simulink model "JumpingHalfLekaSpeedgoat30cm"  (R2024a)
settings: Solver=FixedStepAuto  StartTime=0.0  StopTime=inf  RelTol=1e-3
undefined symbols (not defined in the file): HS, IO291
libraries: aru_toolbox x6, speedgoatlib_IO691 x1, speedgoatlib_IO291 x1, simulink x1
settings Model: Creator=Blue Fifth  LastModifiedBy=user
settings SolverCC: ConcurrentTasks=on  PositivePriorityOrder=on  AutoInsertRateTranBlk=on
settings OptimizationCC: BlockReduction=off  OptimizeBlockIOStorage=off
settings DebuggingCC: TasksWithSamePriorityMsg=none
settings HardwareCC: ProdBitPerLong=64  ProdLongLongMode=on  ProdHWDeviceType=Intel->x86-64 (Linux 64)
settings RTWCC: Description=Speedgoat Real-Time Target Machine  SystemTargetFile=speedgoat.tlc  TemplateMakefile=slrealtime_default_tmf  Toolchain=Simulink Real-Time Toolchain  BuildConfiguration=Faster Runs  CodeExecutionProfiling=on  TargetLang=C++  GPUComputeCapability=3.5
settings SimulinkRealTimeTargetCC: InstructionSetFMA=off  LogToMDFFile=off

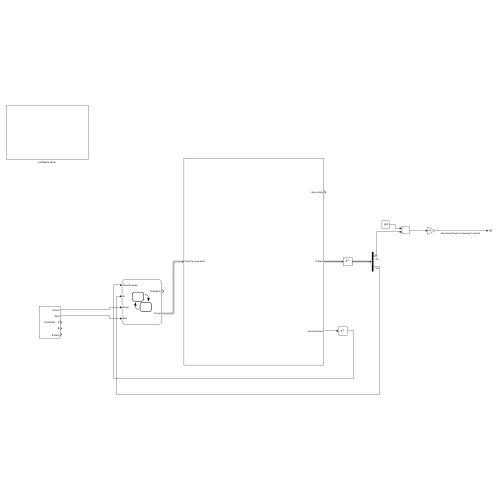
[thumbnail: Simulink's stored preview of the top-level diagram]
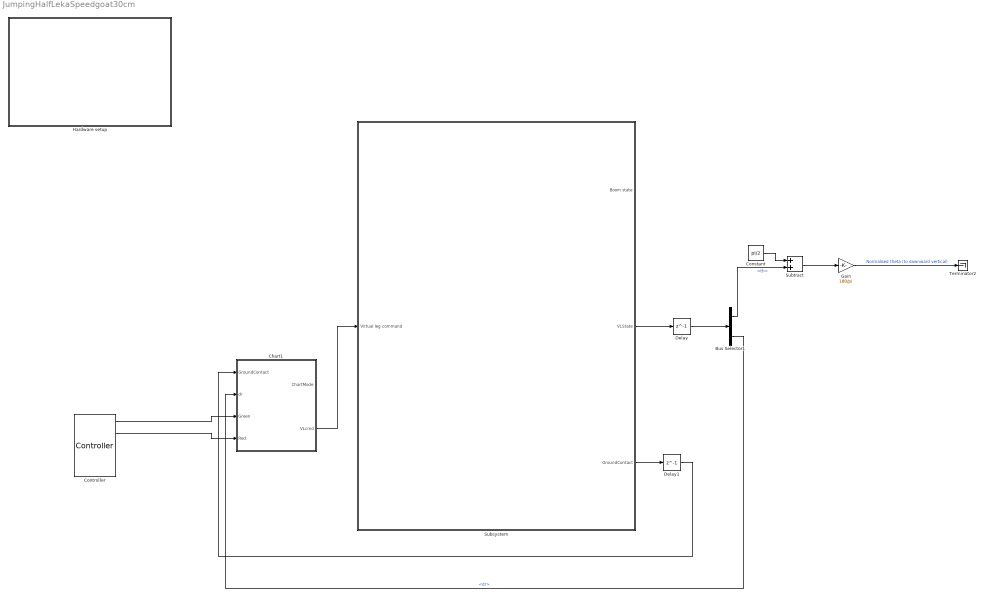
== system JumpingHalfLekaSpeedgoat30cm ==
  Bus Selector1 : BusSelector  OutputSignals=th,dr
  Chart1 : Stateflow chart  TreatAsAtomicUnit=on
  Constant : Constant  Value=pi/2
  Controller : aru_toolbox/Controller
      settings: SourceProductName=ARU Toolbox
  Delay : Delay  DelayLength=1
  Delay1 : Delay  DelayLength=1
  Gain : Gain  Gain=180/pi
  Hardware setup : Subsystem
  Subsystem : Subsystem
  Subtract : Sum
  Terminator2 : Terminator
  wires:
  Controller/1 -> Chart1/3(Green)
  Chart1/2(VLcmd) -> Subsystem/1(Virtual leg command)
  Controller/2 -> Chart1/4(Red)
  Delay1/1 -> Chart1/1(GroundContact)
  Subsystem/2(VLState) -> Delay/1
  Bus Selector1/2 -> Chart1/2(dr)  "<dr>"
  Constant/1 -> Subtract/1
  Subtract/1 -> Gain/1
  Gain/1 -> Terminator2/1  "Normalised theta (to downward vertical)"
  Bus Selector1/1 -> Subtract/2  "<th>"
  Delay/1 -> Bus Selector1/1
  Subsystem/3(GroundContact) -> Delay1/1

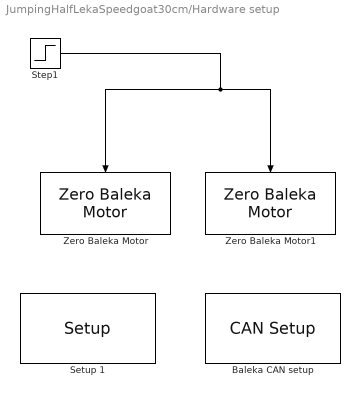
== system JumpingHalfLekaSpeedgoat30cm/Hardware setup ==
  Baleka CAN setup : speedgoatlib_IO691/Legacy/CAN Setup   moduletype=IO691  id=1  pciSlot=-1  chn1=CAN (HS)  chn2=CAN (HS)  chn3=Disabled  chn4=Disabled  initStruct=[]  termStruct=[struct('Channel',1,'Protocol','CAN','BRS',0,'Type','Extended','Identifier',1,'Data',[255, 255, 255, 255, 255, 255, 255, 253],'Pause',0.001), struct('Channel',2,'Protocol','CAN','BRS',0,'Type','Standard','Identifier',2,'Data',[255, 255, 255, 255, 255, 255, 255, 253],'Pause',0.001)]  ArbitrationbdrChn1=1.0 MBaud  ArbitrationManbdrChn1=[2,8,31,8]  FdbdrChn1=1.0 MBaud  FdManbdrChn1=[2,8,31,8]  ArbitrationbdrChn2=1.0 MBaud  ArbitrationManbdrChn2=[2,8,31,8]  FdbdrChn2=1.0 MBaud  FdManbdrChn2=[2,8,31,8]  ArbitrationbdrChn3=1.0 MBaud  ArbitrationManbdrChn3=[2,8,31,8]  FdbdrChn3=5.0 MBaud  FdManbdrChn3=[2,2,5,2]  ArbitrationbdrChn4=1.0 MBaud  ArbitrationManbdrChn4=[2,8,31,8]  FdbdrChn4=5.0 MBaud  FdManbdrChn4=[2,2,5,2]  moduleInitValues=[691 1 -1 -1]
      settings: SourceProductName=IO691
  Setup 1 : speedgoatlib_IO291/Setup   parInternalModuleId=1  parPciSlot=-1  parModuleId=1  parModuleType=IO291-HS  parTtlDoChannels=[]  parTtlDoInitValues=1  parTtlDoReset=1  parTtlDiChannels=[1 2 3 4 5]  parIsolDiChannels=[]  parFetDoChannels=[1 2 3 4 5 6]  parFetDoInitValues=0  parFetDoReset=1
      settings: SourceProductName=IO291
  Step1 : Step  Time=0.3  SampleTime=0
  Zero Baleka Motor : aru_toolbox/Baleka 2.5/Zero Baleka Motor  CAN_ID=1  channel=1
      settings: SourceProductName=ARU Toolbox
  Zero Baleka Motor1 : aru_toolbox/Baleka 2.5/Zero Baleka Motor  CAN_ID=2  channel=1
      settings: SourceProductName=ARU Toolbox
  wires:
  Step1/1 -> Zero Baleka Motor1/Trigger, Zero Baleka Motor/Trigger

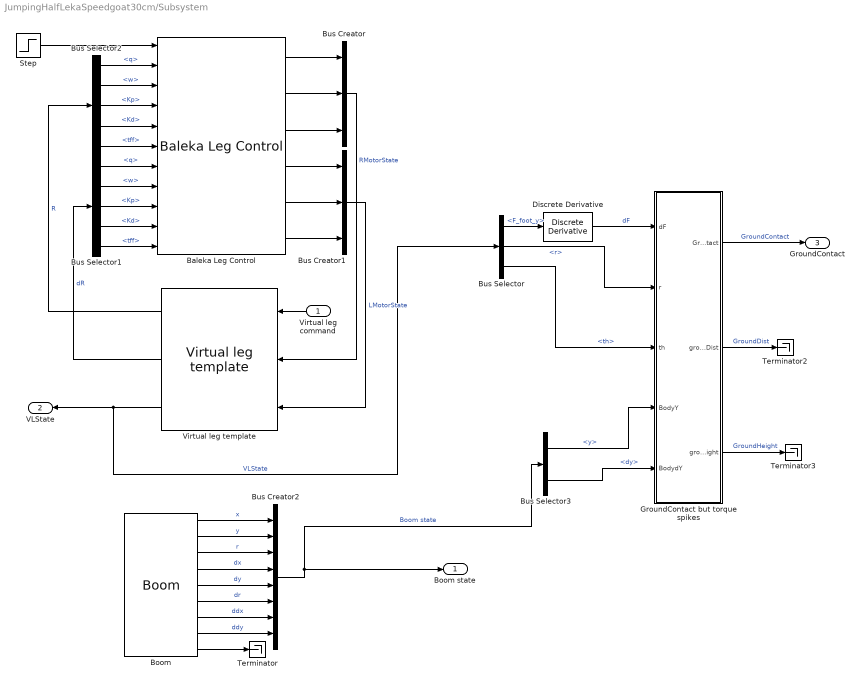
== system JumpingHalfLekaSpeedgoat30cm/Subsystem ==
  Virtual leg command : Inport
  Baleka Leg Control : aru_toolbox/Baleka 2.5/Baleka Leg Control  CAN_ID_L=1  CAN_ID_R=2  channel=1  Comm_freq=1000  enableOffsets=on
      settings: SourceProductName=ARU Toolbox
  Boom : aru_toolbox/Boom  ts=0.001
      settings: SourceProductName=ARU Toolbox
  Bus Creator : BusCreator  Inputs=3  OutDataTypeStr=Bus: MotorState
      settings: InheritFromInputs=off
  Bus Creator1 : BusCreator  Inputs=3  OutDataTypeStr=Bus: MotorState
      settings: InheritFromInputs=off
  Bus Creator2 : BusCreator  Inputs=8  OutDataTypeStr=Bus: BodyState  NonVirtualBus=on
  Bus Selector : BusSelector  OutputSignals=F_foot_y,r,th
  Bus Selector1 : BusSelector  OutputSignals=q,w,Kp,Kd,tff
  Bus Selector2 : BusSelector  OutputSignals=q,w,Kp,Kd,tff
  Bus Selector3 : BusSelector  OutputSignals=y,dy
  Discrete Derivative : simulink/Discrete/Discrete Derivative  gainval=1.0  ICPrevScaledInput=0.0  OutMin=[]  OutMax=[]  OutDataType=fixdt(1, 16)  OutScaling=2^-10  DoSatur=off
  GroundContact but torque spikes : MATLAB Function  TreatAsAtomicUnit=on
  Step : Step  Time=3  SampleTime=0
  Terminator : Terminator
  Terminator2 : Terminator
  Terminator3 : Terminator
  Virtual leg template : aru_toolbox/Baleka 2.5/Virtual leg template  SystemSampleTime=-1  VariantActivationTime=update diagram  AllowFlexibleInterface=on  Latency=0  AutoFrameSizeCalculation=off
      settings: SourceProductName=ARU Toolbox
  Boom state : Outport
  VLState : Outport  Port=2
  GroundContact : Outport  Port=3
  wires:
  Virtual leg template/1 -> Bus Selector2/1  "R"
  Boom/7 -> Bus Creator2/7  "ddx"
  Step/1 -> Baleka Leg Control/1
  Boom/4 -> Bus Creator2/4  "dx"
  Boom/1 -> Bus Creator2/1  "x"
  Boom/2 -> Bus Creator2/2  "y"
  Baleka Leg Control/5 -> Bus Creator1/2
  Bus Selector2/4 -> Baleka Leg Control/5  "<Kd>"
  Baleka Leg Control/3 -> Bus Creator/3
  Boom/6 -> Bus Creator2/6  "dr"
  Baleka Leg Control/2 -> Bus Creator/2
  Baleka Leg Control/6 -> Bus Creator1/3
  Baleka Leg Control/4 -> Bus Creator1/1
  Boom/5 -> Bus Creator2/5  "dy"
  Boom/8 -> Bus Creator2/8  "ddy"
  Bus Selector2/2 -> Baleka Leg Control/3  "<w>"
  Boom/9 -> Terminator/1
  Bus Selector1/1 -> Baleka Leg Control/7  "<q>"
  Bus Selector1/3 -> Baleka Leg Control/9  "<Kp>"
  Bus Creator1/1 -> Virtual leg template/3  "LMotorState"
  Bus Selector1/2 -> Baleka Leg Control/8  "<w>"
  Bus Creator/1 -> Virtual leg template/2  "RMotorState"
  Baleka Leg Control/1 -> Bus Creator/1
  Bus Selector2/1 -> Baleka Leg Control/2  "<q>"
  Virtual leg command/1 -> Virtual leg template/1
  Bus Selector2/3 -> Baleka Leg Control/4  "<Kp>"
  Bus Selector1/4 -> Baleka Leg Control/10  "<Kd>"
  Bus Selector2/5 -> Baleka Leg Control/6  "<tff>"
  Bus Selector1/5 -> Baleka Leg Control/11  "<tff>"
  Boom/3 -> Bus Creator2/3  "r"
  Bus Creator2/1 -> Bus Selector3/1, Boom state/1  "Boom state"
  Virtual leg template/2 -> Bus Selector1/1  "dR"
  Virtual leg template/3 -> Bus Selector/1, VLState/1  "VLState"
  Bus Selector/3 -> GroundContact but torque spikes/3(th)  "<th>"
  Bus Selector3/1 -> GroundContact but torque spikes/4(BodyY)  "<y>"
  Bus Selector3/2 -> GroundContact but torque spikes/5(BodydY)  "<dy>"
  Bus Selector/2 -> GroundContact but torque spikes/2(r)  "<r>"
  Discrete Derivative/1 -> GroundContact but torque spikes/1(dF)  "dF"
  Bus Selector/1 -> Discrete Derivative/1  "<F_foot_y>"
  GroundContact but torque spikes/1(GroundContact) -> GroundContact/1  "GroundContact"
  GroundContact but torque spikes/3(groundHeight) -> Terminator3/1  "GroundHeight"
  GroundContact but torque spikes/2(groundDist) -> Terminator2/1  "GroundDist"

== stateflow chart JumpingHalfLekaSpeedgoat30cm/Chart1 ==
  state Stop
    % Static values
    VLcmd.Tff = 0;
    VLcmd.dth_des =0;
    VLcmd.th_des = -pi/2;
    VLcmd.KPth = 250;
    VLcmd.KDth = 10;
    VLcmd.r_des = 0.45;
    VLcmd.dr_des =0;
    VLcmd.KPr = 1500;
    VLcmd.KDr =50;
    VLcmd.Fff =0;
  state StandUp
    % Static values
    VLcmd.Tff = 0;
    VLcmd.dth_des =0;
    VLcmd.th_des = -pi/2;
    VLcmd.KPth = 50;
    VLcmd.KDth = 5;
    % Gentle stand-up
    VLcmd.r_des = 0.40;
    VLcmd.dr_des =0;
    VLcmd.KPr = 600;
    VLcmd.KDr =50;
    VLcmd.Fff =0;
  state Flight
    % Brace for impact
    VLcmd.r_des = 0.45;
    VLcmd.dr_des =0;
    VLcmd.KPr = 1500;
    VLcmd.KDr =150;
    VLcmd.Fff =0;
    VLcmd.KPth = 350;
    VLcmd.KDth = 10;
  state Contact
    % let spring compress
    VLcmd.r_des = 0.35;
    VLcmd.KPr = 1500;
    VLcmd.KDr =150;
  state Compression
    % let spring compress
  state Thrust
    % Apply upwards thrust force
    VLcmd.r_des = 0.55
    VLcmd.KPr = 1750;
    VLcmd.KDr =0;
    VLcmd.Fff = 0; %Max out upwards thrust
  Stop -> StandUp : [Green>0]
  (default) -> StandUp
  (junction 34) -> Stop
  Compression -> (junction 34) [order 2] : [Red>0]
  Flight -> (junction 34) [order 2] : [Red >0]
  Contact -> (junction 34) [order 2] : [Red>0]
  Thrust -> (junction 34) [order 2] : [Red>0]
  Flight -> Contact [order 1] : [GroundContact]
  StandUp -> Thrust : [Green >0 & after(10, msec)]
  Contact -> Compression [order 1] : [after(100, msec)]
  Thrust -> Flight [order 1] : [~GroundContact]
  Compression -> Thrust [order 1] : [dr<0.01]
  data: ChartMode output Enum: ChartModeType; GroundContact input; dr input; VLcmd output Bus: VLcmd; Green input; Red input

== matlab function JumpingHalfLekaSpeedgoat30cm/Subsystem/GroundContact but torque spikes ==
  data: dF input; r input; th input; GroundContact output; BodyY input; groundDist output; groundHeight output; BodydY input
function [GroundContact, groundDist, groundHeight]  = ImpactTorque(dF,r, th, BodyY, BodydY)
        % need to see how IRL torque spikes work, but we can do a veeery
        % rough guestimate here:
        persistent GroundContactpers;
        persistent GroundHeight;
        if isempty(GroundContactpers)
            GroundContactpers = true;
            GroundHeight = 0;
        end

        if ~GroundContactpers % Impact sensing for gnd
           if (dF>3e4) && (BodydY <0)
            GroundContactpers = true;
            GroundHeight = BodyY  +sin(th)*r; % - 0.004
           end
           groundDist=BodyY + sin(th)*r;
        else 
            % leg length calc for flight
            groundDist = BodyY + sin(th)*r;% - 0.004
            if BodydY >0
                GroundContactpers = ~(groundDist>0.02+GroundHeight);
            end
        end
          
        GroundContact = GroundContactpers;
        groundHeight = GroundHeight;
end
